simulink model "UnitRampResponseModel"  (R2021b)
settings: Solver=VariableStepAuto  StartTime=0.0  StopTime=10.0  RelTol=1e-3
libraries: simulink x1
settings Model: Creator=Lenovo  LastModifiedBy=Lenovo

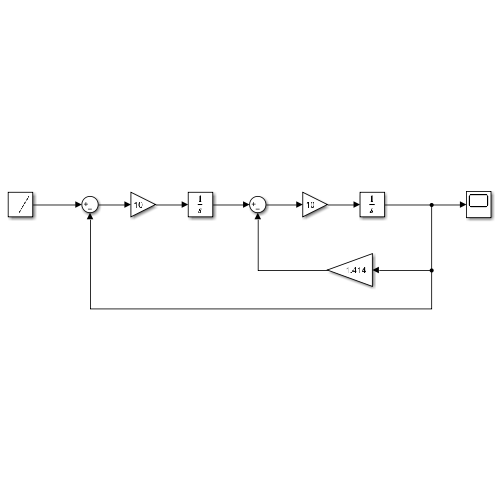
[thumbnail: Simulink's stored preview of the top-level diagram]
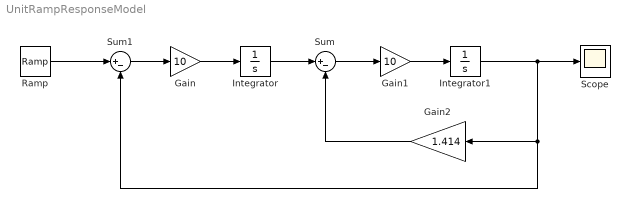
== system UnitRampResponseModel ==
  Gain : Gain  Gain=10
  Gain1 : Gain  Gain=10
  Gain2 : Gain  Gain=1.414
  Integrator : Integrator
  Integrator1 : Integrator
  Ramp : simulink/Sources/Ramp  slope=1  start=0  InitialOutput=0
  Scope : Scope
  Sum : Sum  Inputs=|+-
  Sum1 : Sum  Inputs=|+-
  wires:
  Integrator/1 -> Sum/1
  Gain/1 -> Integrator/1
  Sum/1 -> Gain1/1
  Sum1/1 -> Gain/1
  Gain1/1 -> Integrator1/1
  Gain2/1 -> Sum/2
  Integrator1/1 -> Scope/1, Sum1/2, Gain2/1
  Ramp/1 -> Sum1/1
